simulink model "brush_pid"  (R2013a)
settings: Solver=ode45  StartTime=0.0  StopTime=2.0  RelTol=1e-3
libraries: powerlib x15, simulink x3, electricdrivelib x2
settings Model: Creator=hp  LastModifiedBy=hp

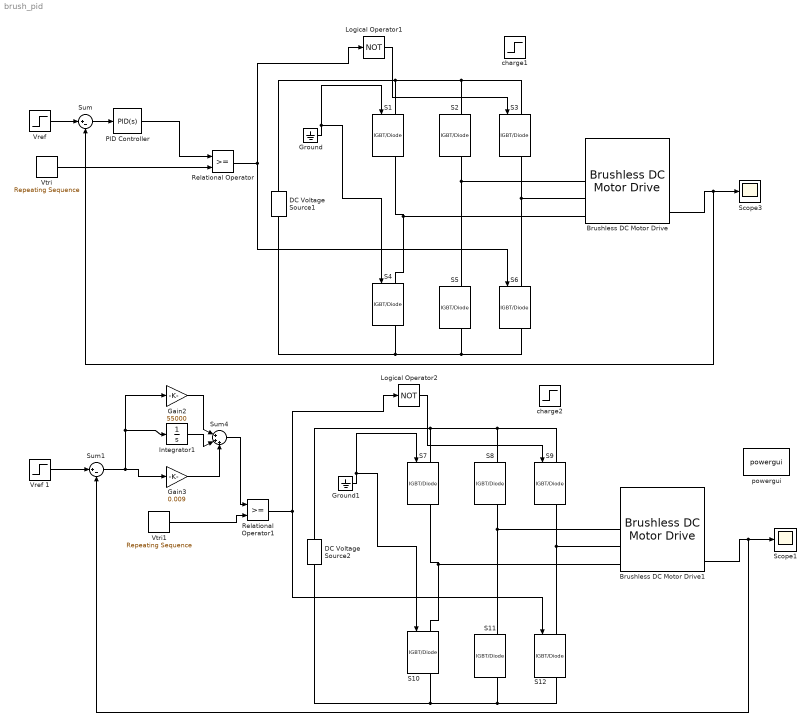
== system brush_pid ==
  Brushless DC Motor Drive : electricdrivelib/AC drives/Brushless DC Motor Drive  showMaskWarnings=on  AverageValue=off  MechanicalLoad=Torque Tm  driveType=AC7
  Brushless DC Motor Drive1 : electricdrivelib/AC drives/Brushless DC Motor Drive  showMaskWarnings=on  AverageValue=off  MechanicalLoad=Torque Tm  driveType=AC7
  DC Voltage Source1 : powerlib/Electrical Sources/DC Voltage Source  Amplitude=240  Measurements=None
  DC Voltage Source2 : powerlib/Electrical Sources/DC Voltage Source  Amplitude=240  Measurements=None
  Gain2 : Gain  Gain=55000
  Gain3 : Gain  Gain=0.009
  Ground : Ground
  Ground1 : Ground
  Integrator1 : Integrator  InitialCondition=11
  Logical Operator1 : Logic  Operator=NOT  AllPortsSameDT=off  OutDataTypeStr=boolean
  Logical Operator2 : Logic  Operator=NOT  AllPortsSameDT=off  OutDataTypeStr=boolean
  PID Controller : simulink/Continuous/PID Controller  Controller=PID  TimeDomain=Continuous-time  SampleTime=1  IntegratorMethod=Forward Euler  FilterMethod=Forward Euler  Form=Parallel  P=55000  I=11  D=0.009  N=100  InitialConditionSource=internal  InitialConditionForIntegrator=0  InitialConditionForFilter=0  ExternalReset=none  LimitOutput=off  UpperSaturationLimit=inf  LowerSaturationLimit=-inf  LinearizeAsGain=on  AntiWindupMode=none  Kb=1  TrackingMode=off  Kt=1  PParamMin=[]  PParamMax=[]  IParamMin=[]  IParamMax=[]  DParamMin=[]  DParamMax=[]  NParamMin=[]  NParamMax=[]  KbParamMin=[]  KbParamMax=[]  KtParamMin=[]  KtParamMax=[]  POutMin=[]  POutMax=[]  IOutMin=[]  IOutMax=[]  DOutMin=[]  DOutMax=[]  NOutMin=[]  NOutMax=[]  KbOutMin=[]  KbOutMax=[]  KtOutMin=[]  KtOutMax=[]  IntegratorOutMin=[]  IntegratorOutMax=[]  FilterOutMin=[]  FilterOutMax=[]  SumOutMin=[]  SumOutMax=[]  SumI1OutMin=[]  SumI1OutMax=[]  SumI2OutMin=[]  SumI2OutMax=[]  SumI3OutMin=[]  SumI3OutMax=[]  SumDOutMin=[]  SumDOutMax=[]  SaturationOutMin=[]  SaturationOutMax=[]  IntegratorContinuousStateAttributes=''  IntegratorStateMustResolveToSignalObject=off  IntegratorRTWStateStorageClass=Auto  FilterContinuousStateAttributes=''  FilterStateMustResolveToSignalObject=off  FilterRTWStateStorageClass=Auto
  Relational Operator : RelationalOperator  OutDataTypeStr=boolean
  Relational Operator1 : RelationalOperator  OutDataTypeStr=boolean
  S{1..12} (12 alike) : powerlib/Power Electronics/IGBT//Diode  Ron=1e-3  Rs=1e5  Cs=inf  Measurements=on
  Scope1 : Scope
      settings: SaveName=IC1
  Scope3 : Scope
      settings: SaveName=IC
  Sum : Sum  Inputs=|+-
  Sum1 : Sum  Inputs=|+-
  Sum4 : Sum  Inputs=|+++
  "Vref " : Step  Time=0  After=150  SampleTime=0
  Vref 1 : Step  Time=0  After=150  SampleTime=0
  Vtri : simulink/Sources/Repeating Sequence  rep_seq_t=[0 (1/2) 1]*0.001  rep_seq_y="[-1  1 -1] *240"
  Vtri1 : simulink/Sources/Repeating Sequence  rep_seq_t=[0 (1/2) 1]*0.001  rep_seq_y="[-1  1 -1] *240"
  charge1 : Step  Time=0.1  After=0.1  SampleTime=0
  charge2 : Step  Time=0.1  After=0.1  SampleTime=0
  powergui : powerlib/powergui  Priority=1  SimulationMode=Discrete  SolverType=Tustin  SampleTime=1e-6  frequency=60  SPID=off  DisableSnubberDevices=off  DisableRonSwitches=off  DisableVfSwitches=off  SwTol=0  Interpol=off  DisplayEquations=off  frequencyindice=0  Pbase=100e6  ErrMax=1e-4  Iterations=50  UnitsV=kV  UnitsW=MW  FunctionMessages=off  echomessages=off  HookPort=off  EnableUseOfTLC=off  x0status=blocks  RestoreLinks=warning  ResistiveCurrentMeasurement=off  Frange=[0:2:500]  Ylog=off  Xlog=on  ShowGrid=off  save=off  variable=ZData  ZoomFFT=off  StartTime=0.0  cycles=1  DisplayStyle=1  fundamental=60  FreqAxis=off  MaxFrequency=1000  frequencyindicesteady=1  RmsSteady=1  display=off  Ts=0  methode=off
  wires:
  Vtri/1 -> Relational Operator/2
  Relational Operator/1 -> S6/1, Logical Operator1/1
  Brushless DC Motor Drive/4 -> Sum/2, Scope3/1
  Logical Operator1/1 -> S3/1
  Ground/1 -> S4/1, S1/1
  "Vref "/1 -> Sum/1
  Sum/1 -> PID Controller/1
  Vtri1/1 -> Relational Operator1/2
  Relational Operator1/1 -> S12/1, Logical Operator2/1
  Brushless DC Motor Drive1/4 -> Sum1/2, Scope1/1
  Logical Operator2/1 -> S9/1
  Ground1/1 -> S10/1, S7/1
  Vref 1/1 -> Sum1/1
  Sum1/1 -> Gain3/1, Integrator1/1, Gain2/1
  Gain2/1 -> Sum4/1
  Integrator1/1 -> Sum4/2
  Gain3/1 -> Sum4/3
  Sum4/1 -> Relational Operator1/1
  PID Controller/1 -> Relational Operator/1
  connections:
  Brushless DC Motor Drive/LConn2 -- S3/RConn1 -- S6/LConn1
  DC Voltage Source1/LConn1 -- S4/RConn1 -- S5/RConn1 -- S6/RConn1
  S2/LConn1 -- S3/LConn1 -- DC Voltage Source1/RConn1 -- S1/LConn1
  Brushless DC Motor Drive/LConn3 -- S1/RConn1 -- S4/LConn1
  Brushless DC Motor Drive/LConn1 -- S2/RConn1 -- S5/LConn1
  Brushless DC Motor Drive1/LConn2 -- S9/RConn1 -- S12/LConn1
  S12/RConn1 -- S11/RConn1 -- S10/RConn1 -- DC Voltage Source2/LConn1
  S7/LConn1 -- DC Voltage Source2/RConn1 -- S9/LConn1 -- S8/LConn1
  Brushless DC Motor Drive1/LConn3 -- S7/RConn1 -- S10/LConn1
  Brushless DC Motor Drive1/LConn1 -- S8/RConn1 -- S11/LConn1
